simulink model "BLDC_Control"  (R2024b)
settings: Solver=VariableStepAuto  StartTime=0.0  StopTime=15  RelTol=1e-3
values from neighbouring files (symbols this model uses):
  b_eq = b_l*(1/r)^2+b_m    (= 2.36823386114e-05)    [Parametros.m]
  c_pitch = cos(pitch)    [Parametros.m]
  J_eq = J_l*(1/r)^2+J_m    [Parametros.m]
  J_eq_nom = 0.5*(J_eq(1)+J_eq(2))    [Parametros.m]
  K_e = 0.0217    [Parametros.m]
  k_l = m*g*l_cm+m_l*g*l_l    [Parametros.m]
  K_t = 21.7e-3    (= 0.0217)    [Parametros.m]
  Kd_m = J_eq(2)*n*w_pos    [Parametros.m]
  ke_int = 32768000000    [Parametros.m]
  ke_tita = 9600    [Parametros.m]
  ke_w = 30720000    [Parametros.m]
  Ki_m = J_eq(2)*w_pos^3    [Parametros.m]
  Kp_m = J_eq(2)*n*w_pos^2-b_eq    [Parametros.m]
  L_s = 0.113e-3    (= 0.000113)    [Parametros.m]
  p = 7    [Parametros.m]
  psi_m = K_e/(1.5*p)    (= 0.00206666666667)    [Parametros.m]
  r = 156    [Parametros.m]
  R_s = 0.196    [Parametros.m]
  s_pitch = sin(pitch)    [Parametros.m]
  s_roll = sin(roll)    [Parametros.m]
  U_d = 18    [Parametros.m]
libraries: eePwmGenerator x1, spsTriangleGeneratorLib x1
settings Model: Creator=ribei  LastModifiedBy=ribei

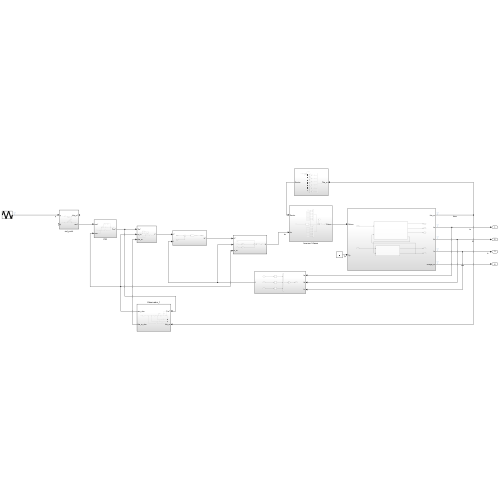
[thumbnail: Simulink's stored preview of the top-level diagram]
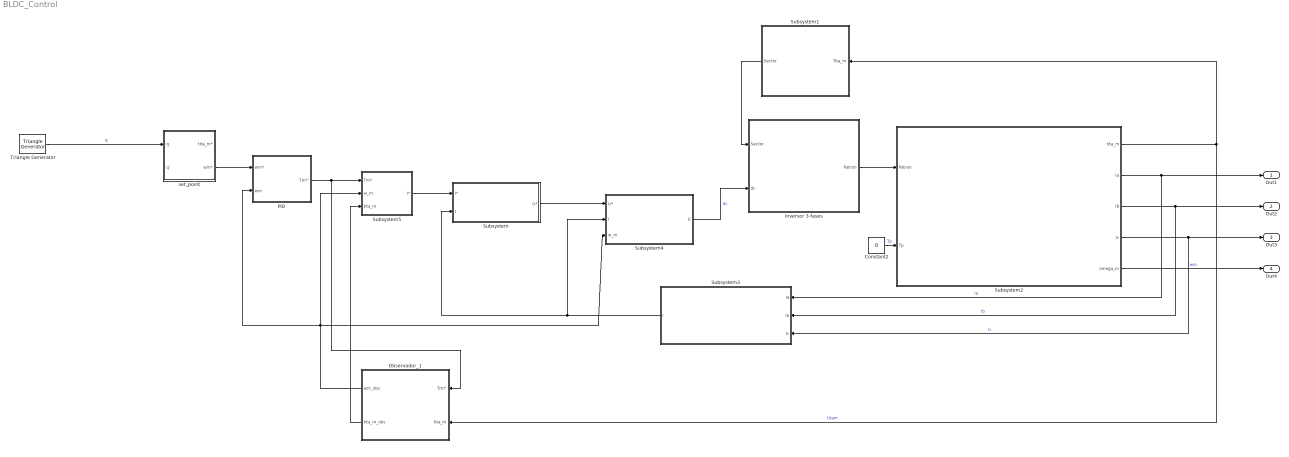
== system BLDC_Control ==
  Constant2 : Constant  Value=0
  Inversor 3-fases : Subsystem
  Observador_1 : Subsystem
  PID : Subsystem
  Subsystem : Subsystem
  Subsystem1 : Subsystem
  Subsystem2 : Subsystem
  Subsystem3 : Subsystem
  Subsystem4 : Subsystem
  Subsystem5 : Subsystem
  Triangle Generator : spsTriangleGeneratorLib/Triangle Generator  Freq=1  Phase=90  Ts=0
  set_point : Subsystem
  Out1 : Outport
  Out2 : Outport  Port=2
  Out3 : Outport  Port=3
  Out4 : Outport  Port=4
  wires:
  Subsystem1/1(Sector) -> Inversor 3-fases/1(Sector)
  Subsystem2/1(tita_m) -> Observador_1/2(tita_m), Subsystem1/1(Tita_m)  "titam"
  Subsystem2/5(omega_m) -> Out4/1  "wm"
  Subsystem2/4(Ic) -> Subsystem3/3(Ic), Out3/1  "Ic"
  Inversor 3-fases/1(Patron) -> Subsystem2/1(Patron)
  Subsystem2/2(Ia) -> Subsystem3/1(Ia), Out1/1  "Ia"
  Constant2/1 -> Subsystem2/2(Tp)  "Tp"
  Subsystem2/3(Ib) -> Subsystem3/2(Ib), Out2/1  "Ib"
  Subsystem4/1(U) -> Inversor 3-fases/2(dc)  "dc"
  set_point/2(wm*) -> PID/1(wm*)
  Triangle Generator/1 -> set_point/1(q)  "q"
  PID/1(Tm*') -> Observador_1/1(Tm*'), Subsystem5/1(Tm*)
  Observador_1/1(wm_obs) -> Subsystem5/2(w_m), Subsystem4/3(w_m), PID/2(wm)
  Subsystem/1(U*) -> Subsystem4/1(U*)
  Subsystem3/1(I) -> Subsystem4/2(I), Subsystem/2(I)
  Subsystem5/1(I*) -> Subsystem/1(I*)
  Observador_1/2(tita_m_obs) -> Subsystem5/3(tita_m)

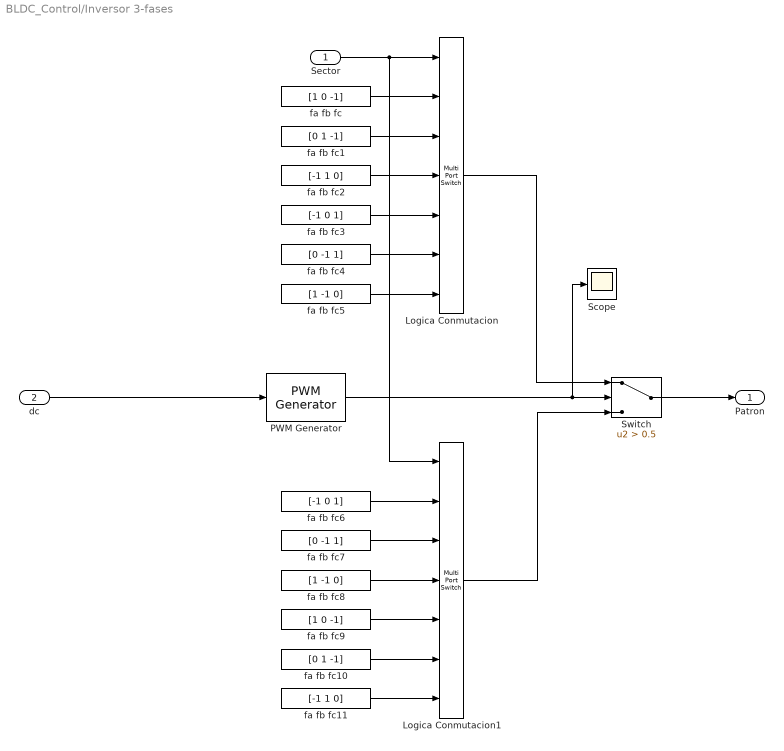
== system BLDC_Control/Inversor 3-fases ==
  Sector : Inport
  dc : Inport  Port=2
  Logica Conmutacion : MultiPortSwitch  Inputs=6  DiagnosticForDefault=None  SaturateOnIntegerOverflow=off  InputSameDT=off
  Logica Conmutacion1 : MultiPortSwitch  Inputs=6  DiagnosticForDefault=None  SaturateOnIntegerOverflow=off  InputSameDT=off
  PWM Generator : eePwmGenerator/PWM Generator  CarrCount=Up  Tper=0.001  Tdelay=0  Ts=5e-5
  Scope : Scope
  Switch : Switch  Criteria=u2 > Threshold  Threshold=0.5  SaturateOnIntegerOverflow=off  InputSameDT=off
  fa fb fc : Constant  Value=[1 0 -1]
  fa fb fc1 : Constant  Value=[0 1 -1]
  fa fb fc10 : Constant  Value=[0 1 -1]
  fa fb fc11 : Constant  Value=[-1 1 0]
  fa fb fc2 : Constant  Value=[-1 1 0]
  fa fb fc3 : Constant  Value=[-1 0 1]
  fa fb fc4 : Constant  Value=[0 -1 1]
  fa fb fc5 : Constant  Value=[1 -1 0]
  fa fb fc6 : Constant  Value=[-1 0 1]
  fa fb fc7 : Constant  Value=[0 -1 1]
  fa fb fc8 : Constant  Value=[1 -1 0]
  fa fb fc9 : Constant  Value=[1 0 -1]
  Patron : Outport
  wires:
  Switch/1 -> Patron/1
  fa fb fc2/1 -> Logica Conmutacion/4
  fa fb fc5/1 -> Logica Conmutacion/7
  Sector/1 -> Logica Conmutacion/1, Logica Conmutacion1/1
  fa fb fc3/1 -> Logica Conmutacion/5
  fa fb fc4/1 -> Logica Conmutacion/6
  fa fb fc1/1 -> Logica Conmutacion/3
  fa fb fc/1 -> Logica Conmutacion/2
  Logica Conmutacion/1 -> Switch/1
  Logica Conmutacion1/1 -> Switch/3
  fa fb fc9/1 -> Logica Conmutacion1/5
  fa fb fc10/1 -> Logica Conmutacion1/6
  fa fb fc11/1 -> Logica Conmutacion1/7
  fa fb fc7/1 -> Logica Conmutacion1/3
  fa fb fc8/1 -> Logica Conmutacion1/4
  fa fb fc6/1 -> Logica Conmutacion1/2
  PWM Generator/1 -> Scope/1, Switch/2
  dc/1 -> PWM Generator/1

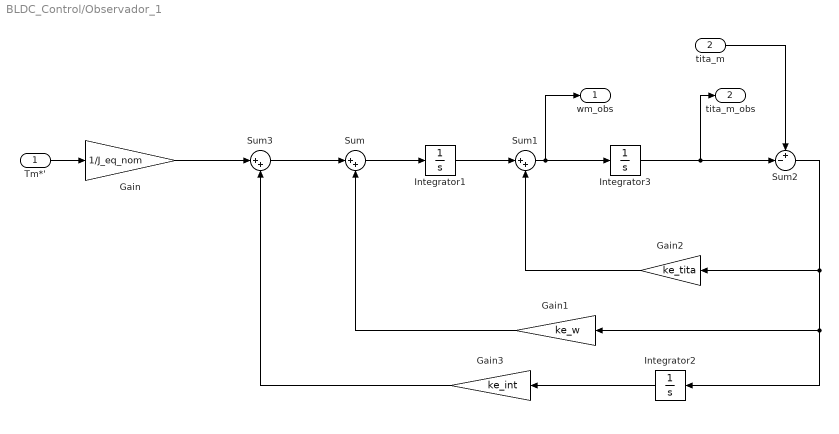
== system BLDC_Control/Observador_1 ==
  Tm*' : Inport
  tita_m : Inport  Port=2
  Gain : Gain  Gain=1/J_eq_nom
  Gain1 : Gain  Gain=ke_w
  Gain2 : Gain  Gain=ke_tita
  Gain3 : Gain  Gain=ke_int
  Integrator1 : Integrator
  Integrator2 : Integrator
  Integrator3 : Integrator
  Sum : Sum  Inputs=|++
  Sum1 : Sum  Inputs=|++
  Sum2 : Sum  Inputs=+-|
  Sum3 : Sum  Inputs=|++
  wm_obs : Outport
  tita_m_obs : Outport  Port=2
  wires:
  Gain2/1 -> Sum1/2
  Tm*'/1 -> Gain/1
  tita_m/1 -> Sum2/1
  Sum2/1 -> Integrator2/1, Gain1/1, Gain2/1
  Gain1/1 -> Sum/2
  Gain3/1 -> Sum3/2
  Sum1/1 -> Integrator3/1, wm_obs/1
  Sum/1 -> Integrator1/1
  Sum3/1 -> Sum/1
  Gain/1 -> Sum3/1
  Integrator1/1 -> Sum1/1
  Integrator2/1 -> Gain3/1
  Integrator3/1 -> Sum2/2, tita_m_obs/1

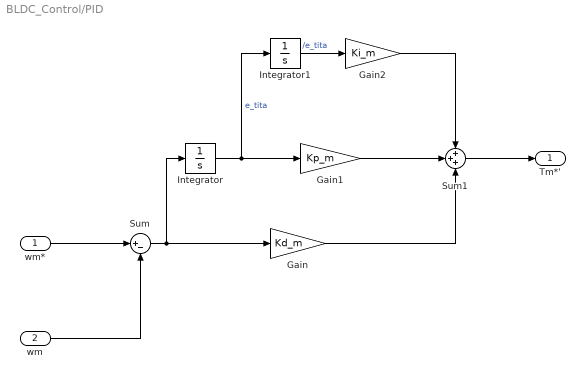
== system BLDC_Control/PID ==
  wm* : Inport
  wm : Inport  Port=2
  Gain : Gain  Gain=Kd_m
  Gain1 : Gain  Gain=Kp_m
  Gain2 : Gain  Gain=Ki_m
  Integrator : Integrator
  Integrator1 : Integrator
  Sum : Sum  Inputs=|+-
  Sum1 : Sum  Inputs=+++
  Tm*' : Outport
  wires:
  Gain2/1 -> Sum1/1
  Gain/1 -> Sum1/3
  Gain1/1 -> Sum1/2
  Sum1/1 -> Tm*'/1
  wm/1 -> Sum/2
  Integrator/1 -> Gain1/1, Integrator1/1  "e_tita"
  Integrator1/1 -> Gain2/1  "/e_tita"
  wm*/1 -> Sum/1
  Sum/1 -> Gain/1, Integrator/1

== system BLDC_Control/Subsystem ==
  I* : Inport
  I : Inport  Port=2
  Gain : Gain  Gain=5000*L_s
  Sum : Sum  Inputs=|+-
  U* : Outport
  wires:
  I*/1 -> Sum/1
  I/1 -> Sum/2
  Gain/1 -> U*/1
  Sum/1 -> Gain/1

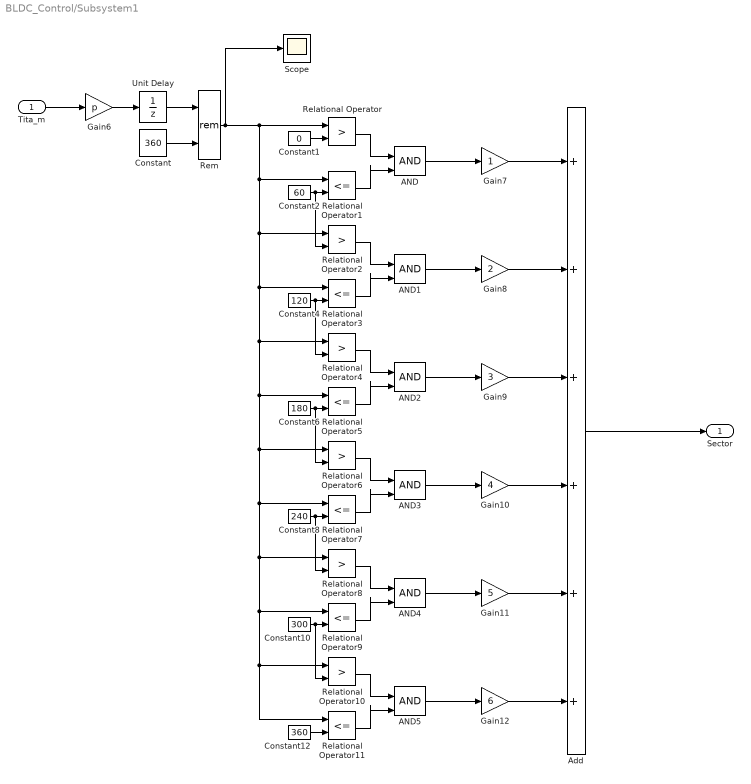
== system BLDC_Control/Subsystem1 ==
  Tita_m : Inport
  AND{,1..5} (6 alike) : Logic  IconShape=distinctive  AllPortsSameDT=off  OutDataTypeStr=boolean
  Add : Sum  Inputs=++++++
  Constant : Constant  Value=360
  Constant1 : Constant  Value=0
  Constant10 : Constant  Value=300
  Constant12 : Constant  Value=360
  Constant2 : Constant  Value=60
  Constant4 : Constant  Value=120
  Constant6 : Constant  Value=180
  Constant8 : Constant  Value=240
  Gain10 : Gain  Gain=4
  Gain11 : Gain  Gain=5
  Gain12 : Gain  Gain=6
  Gain6 : Gain  Gain=p
  Gain7 : Gain
  Gain8 : Gain  Gain=2
  Gain9 : Gain  Gain=3
  Relational Operator{,2,4,6,8,10} (6 alike) : RelationalOperator  Operator=>  OutDataTypeStr=boolean  RndMeth=Simplest  InputSameDT=off
  Relational Operator{1,3,5,7,9,11} (6 alike) : RelationalOperator  Operator=<=  OutDataTypeStr=boolean  RndMeth=Simplest  InputSameDT=off
  Rem : Math  Operator=rem
  Scope : Scope
  Unit Delay : UnitDelay  SampleTime=0.001  HasFrameUpgradeWarning=on
  Sector : Outport
  wires:
  Rem/1 -> Scope/1, Relational Operator/1, Relational Operator1/1, Relational Operator2/1, Relational Operator3/1, Relational Operator4/1, Relational Operator5/1, Relational Operator6/1, Relational Operator7/1, Relational Operator8/1, Relational Operator9/1, Relational Operator10/1, Relational Operator11/1
  AND4/1 -> Gain11/1
  AND1/1 -> Gain8/1
  Relational Operator4/1 -> AND2/1
  Add/1 -> Sector/1
  Gain10/1 -> Add/4
  Relational Operator8/1 -> AND4/1
  Relational Operator3/1 -> AND1/2
  Relational Operator2/1 -> AND1/1
  Gain9/1 -> Add/3
  Constant4/1 -> Relational Operator4/2, Relational Operator3/2
  Constant6/1 -> Relational Operator6/2, Relational Operator5/2
  Gain11/1 -> Add/5
  Constant2/1 -> Relational Operator2/2, Relational Operator1/2
  AND2/1 -> Gain9/1
  Gain7/1 -> Add/1
  Relational Operator5/1 -> AND2/2
  Constant10/1 -> Relational Operator10/2, Relational Operator9/2
  AND/1 -> Gain7/1
  Constant1/1 -> Relational Operator/2
  Relational Operator/1 -> AND/1
  Constant/1 -> Rem/2
  Relational Operator11/1 -> AND5/2
  Constant12/1 -> Relational Operator11/2
  Relational Operator10/1 -> AND5/1
  AND5/1 -> Gain12/1
  Relational Operator9/1 -> AND4/2
  Unit Delay/1 -> Rem/1
  Gain12/1 -> Add/6
  Gain6/1 -> Unit Delay/1
  Tita_m/1 -> Gain6/1
  Constant8/1 -> Relational Operator8/2, Relational Operator7/2
  Relational Operator1/1 -> AND/2
  Relational Operator7/1 -> AND3/2
  AND3/1 -> Gain10/1
  Relational Operator6/1 -> AND3/1
  Gain8/1 -> Add/2

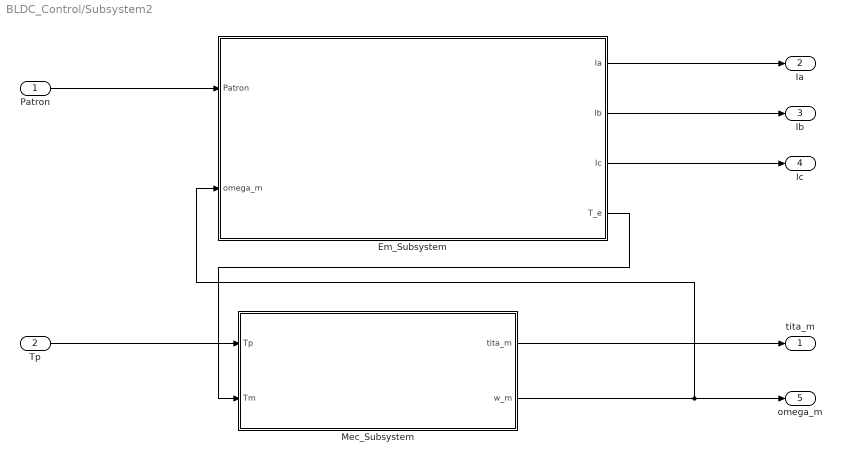
== system BLDC_Control/Subsystem2 ==
  Patron : Inport
  Tp : Inport  Port=2
  Em_Subsystem : Subsystem
  Mec_Subsystem : Subsystem
  tita_m : Outport
  Ia : Outport  Port=2
  Ib : Outport  Port=3
  Ic : Outport  Port=4
  omega_m : Outport  Port=5
  wires:
  Mec_Subsystem/1(tita_m) -> tita_m/1
  Patron/1 -> Em_Subsystem/1(Patron)
  Mec_Subsystem/2(w_m) -> omega_m/1, Em_Subsystem/2(omega_m)
  Em_Subsystem/4(T_e) -> Mec_Subsystem/2(Tm)
  Tp/1 -> Mec_Subsystem/1(Tp)
  Em_Subsystem/1(Ia) -> Ia/1
  Em_Subsystem/3(Ic) -> Ic/1
  Em_Subsystem/2(Ib) -> Ib/1

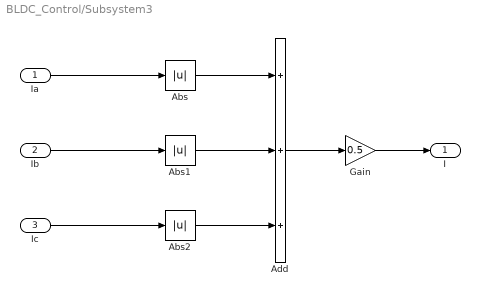
== system BLDC_Control/Subsystem3 ==
  Ia : Inport
  Ib : Inport  Port=2
  Ic : Inport  Port=3
  Abs : Abs  SaturateOnIntegerOverflow=off
  Abs1 : Abs  SaturateOnIntegerOverflow=off
  Abs2 : Abs  SaturateOnIntegerOverflow=off
  Add : Sum  Inputs=+++
  Gain : Gain  Gain=0.5
  I : Outport
  wires:
  Abs/1 -> Add/1
  Abs2/1 -> Add/3
  Abs1/1 -> Add/2
  Ia/1 -> Abs/1
  Ib/1 -> Abs1/1
  Ic/1 -> Abs2/1
  Add/1 -> Gain/1
  Gain/1 -> I/1

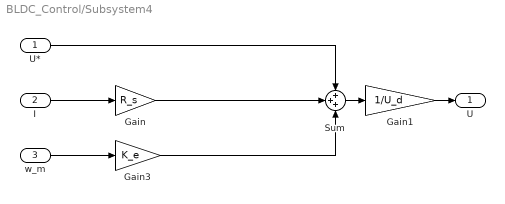
== system BLDC_Control/Subsystem4 ==
  U* : Inport
  I : Inport  Port=2
  w_m : Inport  Port=3
  Gain : Gain  Gain=R_s
  Gain1 : Gain  Gain=1/U_d
  Gain3 : Gain  Gain=K_e
  Sum : Sum  Inputs=+++
  U : Outport
  wires:
  I/1 -> Gain/1
  w_m/1 -> Gain3/1
  Gain/1 -> Sum/2
  U*/1 -> Sum/1
  Gain3/1 -> Sum/3
  Sum/1 -> Gain1/1
  Gain1/1 -> U/1

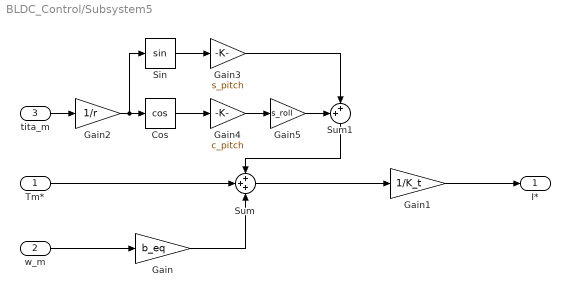
== system BLDC_Control/Subsystem5 ==
  Tm* : Inport
  w_m : Inport  Port=2
  tita_m : Inport  Port=3
  Cos : Trigonometry  Operator=cos
  Gain : Gain  Gain=b_eq
  Gain1 : Gain  Gain=1/K_t
  Gain2 : Gain  Gain=1/r
  Gain3 : Gain  Gain=s_pitch
  Gain4 : Gain  Gain=c_pitch
  Gain5 : Gain  Gain=s_roll
  Sin : Trigonometry
  Sum : Sum  Inputs=+++
  Sum1 : Sum  Inputs=++|
  I* : Outport
  wires:
  w_m/1 -> Gain/1
  Gain/1 -> Sum/3
  Tm*/1 -> Sum/2
  Sum/1 -> Gain1/1
  Gain1/1 -> I*/1
  Gain2/1 -> Cos/1, Sin/1
  tita_m/1 -> Gain2/1
  Cos/1 -> Gain4/1
  Sin/1 -> Gain3/1
  Sum1/1 -> Sum/1
  Gain4/1 -> Gain5/1
  Gain5/1 -> Sum1/1
  Gain3/1 -> Sum1/2

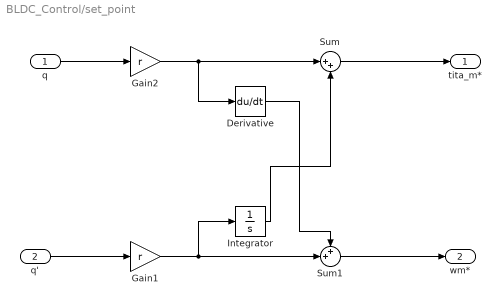
== system BLDC_Control/set_point ==
  q : Inport
  q' : Inport  Port=2
  Derivative : Derivative
  Gain1 : Gain  Gain=r
  Gain2 : Gain  Gain=r
  Integrator : Integrator
  Sum : Sum  Inputs=|++
  Sum1 : Sum  Inputs=++|
  tita_m* : Outport
  wm* : Outport  Port=2
  wires:
  q'/1 -> Gain1/1
  Gain2/1 -> Derivative/1, Sum/1
  Sum/1 -> tita_m*/1
  q/1 -> Gain2/1
  Derivative/1 -> Sum1/1
  Gain1/1 -> Integrator/1, Sum1/2
  Sum1/1 -> wm*/1
  Integrator/1 -> Sum/2

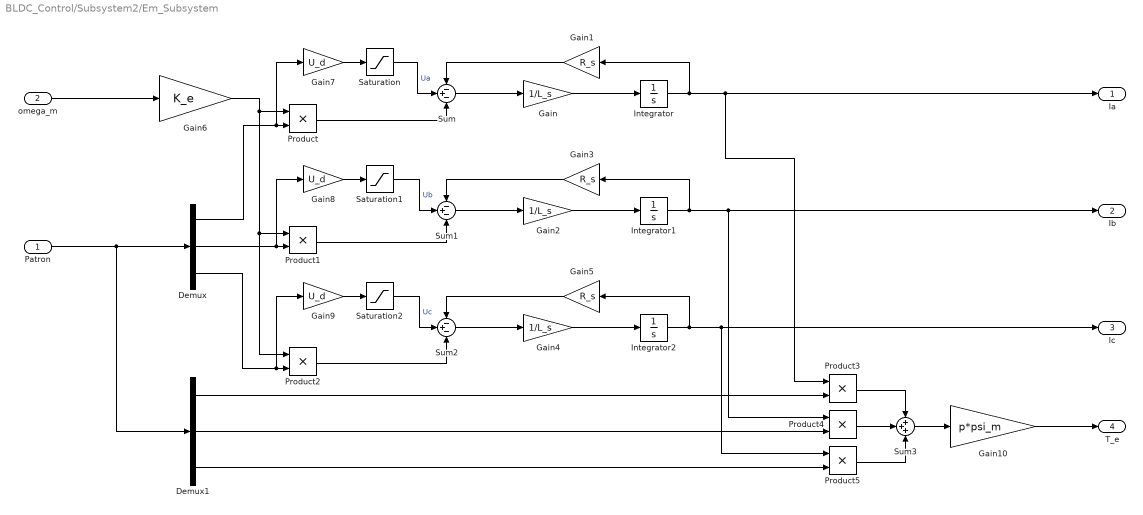
== system BLDC_Control/Subsystem2/Em_Subsystem ==
  Patron : Inport
  omega_m : Inport  Port=2
  Demux : Demux  Outputs=3
  Demux1 : Demux  Outputs=3
  Gain : Gain  Gain=1/L_s
  Gain1 : Gain  Gain=R_s
  Gain10 : Gain  Gain=p*psi_m
  Gain2 : Gain  Gain=1/L_s
  Gain3 : Gain  Gain=R_s
  Gain4 : Gain  Gain=1/L_s
  Gain5 : Gain  Gain=R_s
  Gain6 : Gain  Gain=K_e
  Gain7 : Gain  Gain=U_d
  Gain8 : Gain  Gain=U_d
  Gain9 : Gain  Gain=U_d
  Integrator : Integrator
  Integrator1 : Integrator
  Integrator2 : Integrator
  Product{,1..5} (6 alike) : Product
  Saturation : Saturate  UpperLimit=18  LowerLimit=0
  Saturation1 : Saturate  UpperLimit=18  LowerLimit=0
  Saturation2 : Saturate  UpperLimit=18  LowerLimit=0
  Sum : Sum  Inputs=-+-
  Sum1 : Sum  Inputs=-+-
  Sum2 : Sum  Inputs=-+-
  Sum3 : Sum  Inputs=+++
  Ia : Outport
  Ib : Outport  Port=2
  Ic : Outport  Port=3
  T_e : Outport  Port=4
  wires:
  Gain/1 -> Integrator/1
  Integrator/1 -> Gain1/1, Product3/1, Ia/1
  Sum/1 -> Gain/1
  Gain1/1 -> Sum/1
  Sum1/1 -> Gain2/1
  Gain3/1 -> Sum1/1
  Gain2/1 -> Integrator1/1
  Integrator1/1 -> Product4/1, Ib/1, Gain3/1
  Gain4/1 -> Integrator2/1
  Gain5/1 -> Sum2/1
  Sum2/1 -> Gain4/1
  Integrator2/1 -> Product5/1, Ic/1, Gain5/1
  omega_m/1 -> Gain6/1
  Gain6/1 -> Product2/1, Product1/1, Product/1
  Demux/1 -> Gain7/1, Product/2
  Demux/2 -> Gain8/1, Product1/2
  Demux/3 -> Gain9/1, Product2/2
  Product/1 -> Sum/3
  Product1/1 -> Sum1/3
  Product2/1 -> Sum2/3
  Gain7/1 -> Saturation/1
  Gain8/1 -> Saturation1/1
  Gain9/1 -> Saturation2/1
  Patron/1 -> Demux1/1, Demux/1
  Demux1/1 -> Product3/2
  Demux1/2 -> Product4/2
  Demux1/3 -> Product5/2
  Product3/1 -> Sum3/1
  Product4/1 -> Sum3/2
  Product5/1 -> Sum3/3
  Sum3/1 -> Gain10/1
  Gain10/1 -> T_e/1
  Saturation/1 -> Sum/2  "Ua"
  Saturation1/1 -> Sum1/2  "Ub"
  Saturation2/1 -> Sum2/2  "Uc"

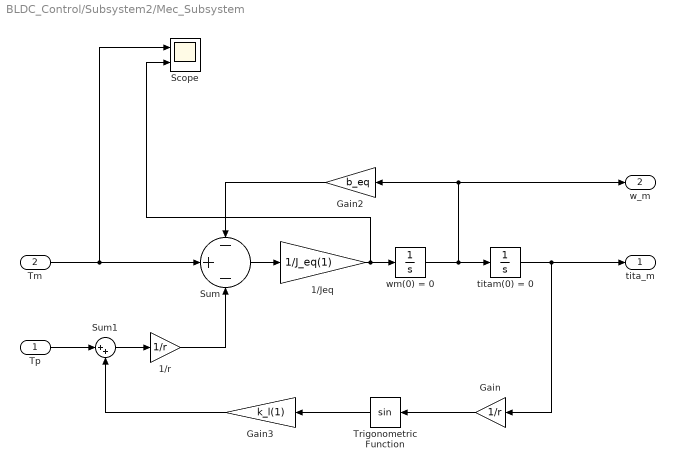
== system BLDC_Control/Subsystem2/Mec_Subsystem ==
  Tp : Inport
  Tm : Inport  Port=2
  1/Jeq : Gain  Gain=1/J_eq(1)
  1/r : Gain  Gain=1/r
  Gain : Gain  Gain=1/r
  Gain2 : Gain  Gain=b_eq
  Gain3 : Gain  Gain=k_l(1)
  Scope : Scope  NumInputPorts=2
  Sum : Sum  Inputs=-+-
  Sum1 : Sum  Inputs=|++
  Trigonometric Function : Trigonometry
  titam(0) = 0 : Integrator
  wm(0) = 0 : Integrator
  tita_m : Outport
  w_m : Outport  Port=2
  wires:
  wm(0) = 0/1 -> Gain2/1, w_m/1, titam(0) = 0/1
  1/r/1 -> Sum/3
  titam(0) = 0/1 -> Gain/1, tita_m/1
  Tp/1 -> Sum1/1
  Sum1/1 -> 1/r/1
  Tm/1 -> Scope/1, Sum/2
  Gain2/1 -> Sum/1
  Sum/1 -> 1/Jeq/1
  Trigonometric Function/1 -> Gain3/1
  1/Jeq/1 -> Scope/2, wm(0) = 0/1
  Gain/1 -> Trigonometric Function/1
  Gain3/1 -> Sum1/2
